simulink model "Step"  (R2023a)
settings: Solver=ode45  StartTime=0.0  StopTime=3.0  MaxStep=0.001  RelTol=1e-6  AbsTol=1e-6
undefined symbols (not defined in the file): B, J, Kp, Kt, Kw, L, R
settings Model: Creator=karteek  LastModifiedBy=karteek
settings DataIOCC: SaveOutput=off  SignalLogging=off  DSMLogging=off  SaveTime=off  ReturnWorkspaceOutputs=off

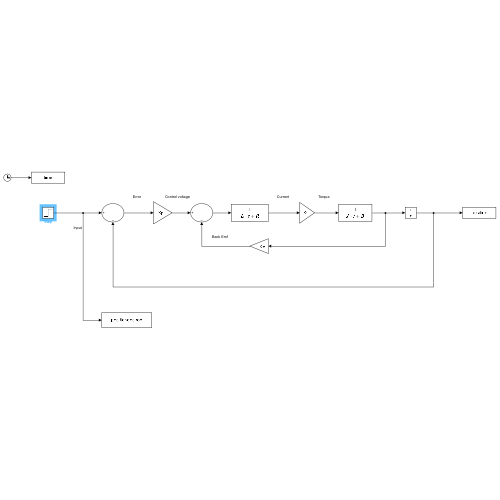
[thumbnail: Simulink's stored preview of the top-level diagram]
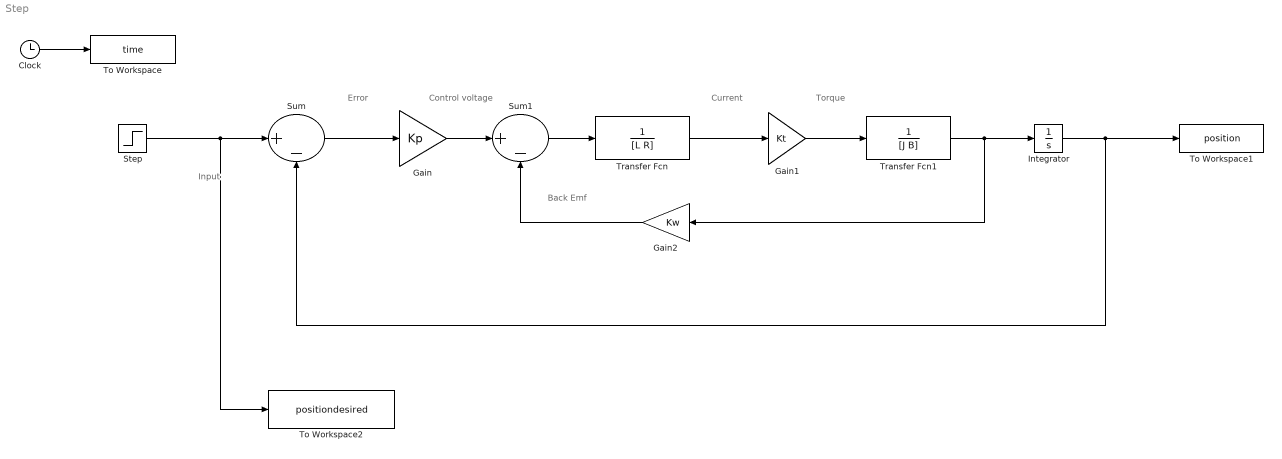
== system Step ==
  note: Torque
  note: Current
  note: Back Emf
  note: Control voltage
  note: Error
  note: Input
  Clock : Clock
  Gain : Gain  Gain=Kp
  Gain1 : Gain  Gain=Kt
  Gain2 : Gain  Gain=Kw
  Integrator : Integrator
  Step : Step  After=pi/2  SampleTime=0
  Sum : Sum  Inputs=|+-
  Sum1 : Sum  Inputs=|+-
  To Workspace : ToWorkspace  VariableName=time  SampleTime=-1
  To Workspace1 : ToWorkspace  VariableName=position  SampleTime=-1
  To Workspace2 : ToWorkspace  VariableName=positiondesired  SampleTime=-1
  Transfer Fcn : TransferFcn  Denominator=[L R]
  Transfer Fcn1 : TransferFcn  Denominator=[J B]
  wires:
  Sum/1 -> Gain/1
  Gain/1 -> Sum1/1
  Sum1/1 -> Transfer Fcn/1
  Transfer Fcn/1 -> Gain1/1
  Gain1/1 -> Transfer Fcn1/1
  Gain2/1 -> Sum1/2
  Transfer Fcn1/1 -> Gain2/1, Integrator/1
  Clock/1 -> To Workspace/1
  Step/1 -> Sum/1, To Workspace2/1
  Integrator/1 -> Sum/2, To Workspace1/1
